simulink model "yobuto_test_ros"  (R2018b)
settings: Solver=FixedStepAuto  StartTime=0.0  StopTime=inf  RelTol=1e-3
libraries: robotlib x7
settings Model: Creator=kika  LastModifiedBy=kika

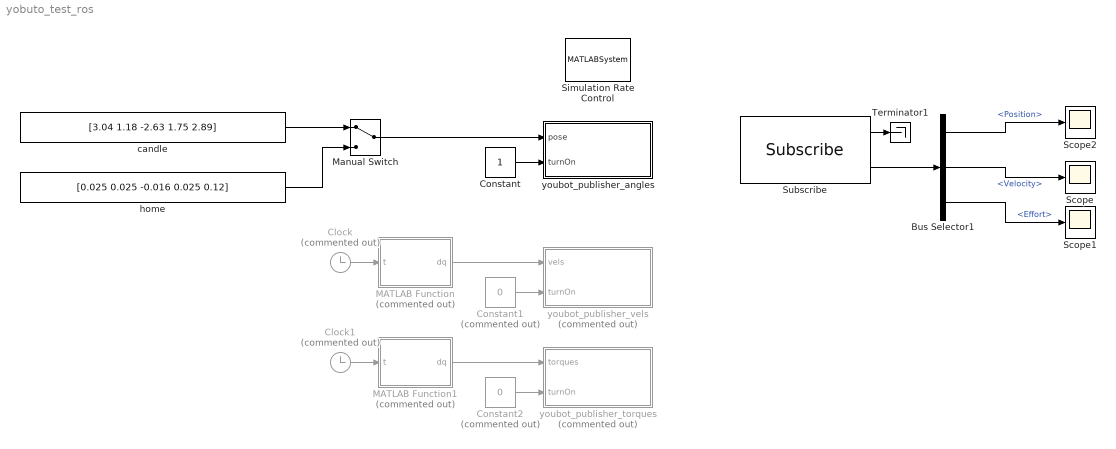
== system yobuto_test_ros ==
  Bus Selector1 : BusSelector  OutputSignals=Position,Velocity,Effort
  Clock : Clock  Commented=on
  Clock1 : Clock  Commented=on
  Constant : Constant
  Constant1 : Constant  Commented=on  Value=0
  Constant2 : Constant  Commented=on  Value=0
  MATLAB Function : MATLAB Function  Commented=on  TreatAsAtomicUnit=on
  MATLAB Function1 : MATLAB Function  Commented=on  TreatAsAtomicUnit=on
  Manual Switch : ManualSwitch
  Scope : Scope
  Scope1 : Scope
  Scope2 : Scope
  Simulation Rate Control : MATLABSystem  System=ExampleHelperSimulationRateControl  SampleTime=0.05
      mask Type: ExampleHelperSimulationRateControl
      mask Display: disp('Rate Control');
  Subscribe : robotlib/Subscribe  topicSource=Select from ROS network  topic=/joint_states  messageType=sensor_msgs/JointState  sampleTime=-1  messageQueueLength=1
      settings: SourceProductBaseCode=RO
  Terminator1 : Terminator
  candle : Constant  Value=[3.04 1.18 -2.63 1.75 2.89]
  home : Constant  Value=[0.025 0.025 -0.016 0.025 0.12]
  "youbot_publisher_angles " : Subsystem
  youbot_publisher_torques : Subsystem  Commented=on
  youbot_publisher_vels : Subsystem  Commented=on
  wires:
  Subscribe/2 -> Bus Selector1/1
  Subscribe/1 -> Terminator1/1
  Bus Selector1/1 -> Scope2/1  "<Position>"
  Constant/1 -> "youbot_publisher_angles "/2(turnOn)
  candle/1 -> Manual Switch/1
  Manual Switch/1 -> "youbot_publisher_angles "/1(pose)
  home/1 -> Manual Switch/2
  Bus Selector1/2 -> Scope/1  "<Velocity>"
  Bus Selector1/3 -> Scope1/1  "<Effort>"
  Constant1/1 -> youbot_publisher_vels/2(turnOn)
  MATLAB Function/1(dq) -> youbot_publisher_vels/1(vels)
  Clock/1 -> MATLAB Function/1(t)
  Constant2/1 -> youbot_publisher_torques/2(turnOn)
  Clock1/1 -> MATLAB Function1/1(t)
  MATLAB Function1/1(dq) -> youbot_publisher_torques/1(torques)

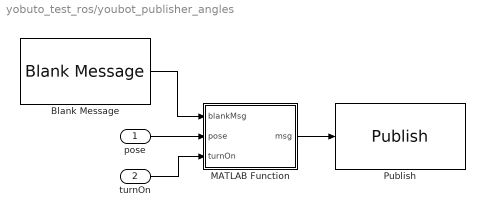
== system yobuto_test_ros/youbot_publisher_angles  ==
  pose : Inport
  turnOn : Inport  Port=2
  Blank Message : robotlib/Blank Message  messageClass=Message  entityType=brics_actuator/JointPositions  messageType=brics_actuator/JointPositions  SampleTime=inf
      settings: SourceProductBaseCode=RO
  MATLAB Function : MATLAB Function  TreatAsAtomicUnit=on
  Publish : robotlib/Publish  topicSource=Select from ROS network  topic=/arm_1/arm_controller/position_command  messageType=brics_actuator/JointPositions  messageQueueLength=1
      settings: SourceProductBaseCode=RO
  wires:
  MATLAB Function/1(msg) -> Publish/1
  pose/1 -> MATLAB Function/2(pose)
  Blank Message/1 -> MATLAB Function/1(blankMsg)
  turnOn/1 -> MATLAB Function/3(turnOn)

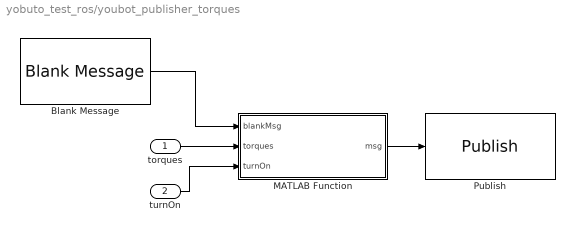
== system yobuto_test_ros/youbot_publisher_torques ==
  torques : Inport
  turnOn : Inport  Port=2
  Blank Message : robotlib/Blank Message  messageClass=Message  entityType=brics_actuator/JointTorques  messageType=brics_actuator/JointTorques  SampleTime=inf
      settings: SourceProductBaseCode=RO
  MATLAB Function : MATLAB Function  TreatAsAtomicUnit=on
  Publish : robotlib/Publish  topicSource=Select from ROS network  topic=/arm_1/arm_controller/torques_command  messageType=brics_actuator/JointTorques  messageQueueLength=1
      settings: SourceProductBaseCode=RO
  wires:
  MATLAB Function/1(msg) -> Publish/1
  torques/1 -> MATLAB Function/2(torques)
  Blank Message/1 -> MATLAB Function/1(blankMsg)
  turnOn/1 -> MATLAB Function/3(turnOn)

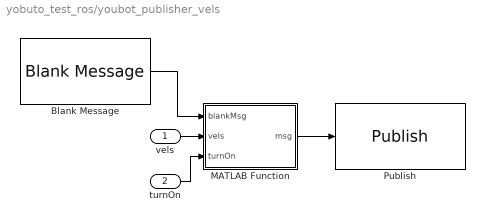
== system yobuto_test_ros/youbot_publisher_vels ==
  vels : Inport
  turnOn : Inport  Port=2
  Blank Message : robotlib/Blank Message  messageClass=Message  entityType=brics_actuator/JointVelocities  messageType=brics_actuator/JointVelocities  SampleTime=inf
      settings: SourceProductBaseCode=RO
  MATLAB Function : MATLAB Function  TreatAsAtomicUnit=on
  Publish : robotlib/Publish  topicSource=Select from ROS network  topic=/arm_1/arm_controller/velocity_command  messageType=brics_actuator/JointVelocities  messageQueueLength=1
      settings: SourceProductBaseCode=RO
  wires:
  MATLAB Function/1(msg) -> Publish/1
  vels/1 -> MATLAB Function/2(vels)
  Blank Message/1 -> MATLAB Function/1(blankMsg)
  turnOn/1 -> MATLAB Function/3(turnOn)

== matlab function yobuto_test_ros/youbot_publisher_angles /MATLAB Function ==
  data: blankMsg input; msg output Bus: SL_Bus_test_ros_brics_actuator_JointPositions; pose input; turnOn input
function msg = setPose(blankMsg, pose, turnOn)
    persistent Sec
    if isempty(Sec)
        Sec = 0;
    end
    if turnOn

        n = 5;
        uri = 'arm_joint_';
        unit = 'rad';

        blankMsg.Positions_SL_Info.CurrentLength = uint32(n);

        for i = 1:n
            %bmsg.Positions(i).TimeStamp.Sec = Sec;   

            strLength = length(uri) + 1;    % plus index of joint
            blankMsg.Positions(i).JointUri(1:strLength) = [uint8(uri), uint8(i + 48)]; % shift in ascii table for number '0'
            blankMsg.Positions(i).JointUri_SL_Info.CurrentLength = uint32(strLength);

            strLength = length(unit);
            blankMsg.Positions(i).Unit(1:strLength) = uint8(unit);
            blankMsg.Positions(i).Unit_SL_Info.CurrentLength = uint32(strLength);

            blankMsg.Positions(i).Value = pose(i);
        end

        
        
        Sec = Sec + 1;
    end
    msg = blankMsg;
end

== matlab function yobuto_test_ros/youbot_publisher_vels/MATLAB Function ==
  data: blankMsg input; msg output Bus: SL_Bus_test_ros_brics_actuator_JointVelocities; vels input; turnOn input
function msg = setVels(blankMsg, vels, turnOn)
    persistent Sec
    if isempty(Sec)
        Sec = 0;
    end
    
    n = 5;
    uri = 'arm_joint_';
    unit = 's^-1 rad';

    blankMsg.Velocities_SL_Info.CurrentLength = uint32(n);

    for i = 1:n
        %bmsg.Velocities(i).TimeStamp.Sec = Sec;   

        strLength = length(uri) + 1;    % plus index of joint
        blankMsg.Velocities(i).JointUri(1:strLength) = [uint8(uri), uint8(i + 48)]; % shift in ascii table for number '0'
        blankMsg.Velocities(i).JointUri_SL_Info.CurrentLength = uint32(strLength);

        strLength = length(unit);
        blankMsg.Velocities(i).Unit(1:strLength) = uint8(unit);
        blankMsg.Velocities(i).Unit_SL_Info.CurrentLength = uint32(strLength);

        if turnOn
            blankMsg.Velocities(i).Value = vels(i);
        else
            blankMsg.Velocities(i).Value = 0;
        end
    end
    Sec = Sec + 1;

    msg = blankMsg;
end

== matlab function yobuto_test_ros/youbot_publisher_torques/MATLAB Function ==
  data: blankMsg input; msg output Bus: SL_Bus_test_ros_brics_actuator_JointTorques; torques input; turnOn input
function msg = setTorque(blankMsg, torques, turnOn)
    persistent Sec
    if isempty(Sec)
        Sec = 0;
    end
    
    n = 5;
    uri = 'arm_joint_';
    unit = 'm^2 kg s^-2 rad^-1';

    blankMsg.Torques_SL_Info.CurrentLength = uint32(n);

    for i = 1:n
        %bmsg.Torques(i).TimeStamp.Sec = Sec;   

        strLength = length(uri) + 1;    % plus index of joint
        blankMsg.Torques(i).JointUri(1:strLength) = [uint8(uri), uint8(i + 48)]; % shift in ascii table for number '0'
        blankMsg.Torques(i).JointUri_SL_Info.CurrentLength = uint32(strLength);

        strLength = length(unit);
        blankMsg.Torques(i).Unit(1:strLength) = uint8(unit);
        blankMsg.Torques(i).Unit_SL_Info.CurrentLength = uint32(strLength);

        if turnOn
            blankMsg.Torques(i).Value = torques(i);
        else
            blankMsg.Torques(i).Value = 0;
        end

    end
    Sec = Sec + 1;
    msg = blankMsg;    
end

== matlab function yobuto_test_ros/MATLAB Function ==
  data: t input; dq output
function dq = vels(t)

dq = [0.5 * sin(4*t) 0 0 0 0];

== matlab function yobuto_test_ros/MATLAB Function1 ==
  data: t input; dq output
function dq = vels(t)

dq = [0.5 * sin(4*t) 0 0 0 0];
